simulink model "Z6"  (R2016b)
settings: Solver=VariableStepAuto  StartTime=0.0  StopTime=10  RelTol=1e-3
settings Model: Creator=Milan Sas  LastModifiedBy=Milan Sas

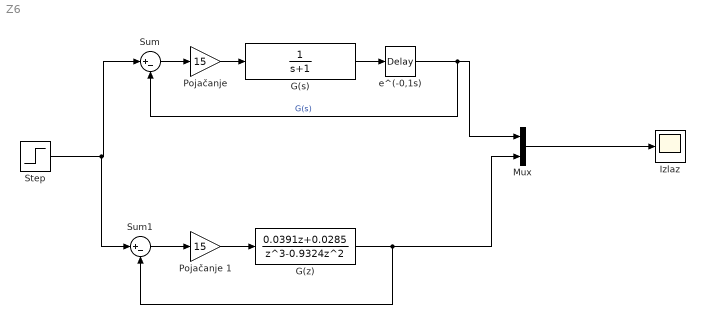
== system Z6 ==
  G(s) : TransferFcn  Denominator=[1 1]
  G(z) : DiscreteTransferFcn  Numerator=[0.0391 0.0285]  Denominator=[1 -0.9324 0 0]  SampleTime=0.07
  Izlaz : Scope
  Mux : Mux  Inputs=2
  Pojačanje : Gain  Gain=15
  Pojačanje 1 : Gain  Gain=15
  Step : Step  SampleTime=0
  Sum : Sum  Inputs=|+-
  Sum1 : Sum  Inputs=|+-
  e^(-0,1s) : TransportDelay  DelayTime=0.1
  wires:
  G(z)/1 -> Sum1/2, Mux/2
  G(s)/1 -> e^(-0,1s)/1
  Step/1 -> Sum1/1, Sum/1
  Mux/1 -> Izlaz/1
  e^(-0,1s)/1 -> Mux/1, Sum/2  "G(s)"
  Sum1/1 -> Pojačanje 1/1
  Pojačanje 1/1 -> G(z)/1
  Pojačanje/1 -> G(s)/1
  Sum/1 -> Pojačanje/1
